simulink model "AGTF30SysDyn_PExPIn"  (R2021b)
settings: Solver=ode4  StartTime=0.0  StopTime=MWS.In.tend  FixedStep=MWS.In.Ts  RelTol=1e-3  EnableMultiTasking=on
model workspace: external: MAT-File (data not in the file)
values from neighbouring files (symbols this model uses):
  MWS = setup_initialize(MWS,startPt,SSsolverSP)    [Setup_Simulation.m]    (also in run_AGTF30e_script.m = Setup_Simulation(inputMethod,MWS.In,filename,Mdl,SSsolverSP,)
undefined symbols (not defined in the file or in its folder): DiscIntNeverNeededParam
libraries: Lib_Solve_ModelSource_TMATS x28, Lib_Cntrl_FirstOrderSensor_TMATS x19, simulink x12, Lib_Cntrl_FirstOrderActuator_TMATS x2, Lib_Cntrl_LimitSelect_TMATS x2, Lib_Solve_OuterLoopIntegrator_TMATS x2, Lib_Cntrl_CorrectedSpeed_TMATS x1, Lib_Solve_IterNRSolverJC_TMATS x1
(part 5 of 6)

== system AGTF30SysDyn_PExPIn/Control System/Wf Controller/Controller/Wf Limit Controllers/Accel Controller ==
  Alt : Inport
  MN : Inport  Port=2
  N1cN : Inport  Port=3
  phiEPT : Inport  Port=4
  phiBoost : Inport  Port=5
  Wfmax : Inport  Port=6
  Wfcmd : Inport  Port=7
  ps3 : Inport  Port=8
  Constant : Constant  Value=MWS.In.Options.WfTransientLogic
  Constant1 : Constant  Value=MWS.In.Options.HybridConfig
  Constant2 : Constant
  Constant3 : Constant  Value=-4*MWS.In.Ts
  Constant4 : Constant  Value=MWS.In.Options.TEEM
  Constant5 : Constant
  Constant6 : Constant  Value=1.1/1.03
  Divide1 : Product  Inputs=**
  Divide2 : Product  Inputs=**
  Divide3 : Product  Inputs=*/
  Divide4 : Product  Inputs=**
  Gain2 : Gain  Gain=MWS.Cntrl.WfCntrl.GenAccel.CeilingMultiplier
  Math Function : Math  SaturateOnIntegerOverflow=on
  Memory : Memory  InitialCondition=MWS.Init.IC.Wf
  Multiport Switch : MultiPortSwitch
  RUSched_Boost : Lookup_n-D  NumberOfTableDimensions=5  BreakpointsForDimension1=MWS.Cntrl.WfCntrl.Accel.Boost.RUsch.N1cN_vec  BreakpointsForDimension2=MWS.Cntrl.WfCntrl.Accel.Boost.RUsch.Alt_vec  BreakpointsForDimension3=MWS.Cntrl.WfCntrl.Accel.Boost.RUsch.MN_vec  BreakpointsForDimension4=MWS.Cntrl.WfCntrl.Accel.Boost.RUsch.phiEPT_vec  BreakpointsForDimension5=MWS.Cntrl.WfCntrl.Accel.Boost.RUsch.phiBoost_vec  Table=MWS.Cntrl.WfCntrl.Accel.Boost.RUsch.RU_array  ExtrapMethod=Clip  InternalRulePriority=Speed  RndMeth=Simplest  InputSameDT=on
      settings: InputPortMap=u0,u1,u2,u3,u4
  RUSched_PEx : Lookup_n-D  NumberOfTableDimensions=4  BreakpointsForDimension1=MWS.Cntrl.WfCntrl.Accel.PEx.RUsch.N1cN_vec  BreakpointsForDimension2=MWS.Cntrl.WfCntrl.Accel.PEx.RUsch.Alt_vec  BreakpointsForDimension3=MWS.Cntrl.WfCntrl.Accel.PEx.RUsch.MN_vec  BreakpointsForDimension4=MWS.Cntrl.WfCntrl.Accel.PEx.RUsch.phiEPT_vec  Table=MWS.Cntrl.WfCntrl.Accel.PEx.RUsch.RU_array  ExtrapMethod=Clip  InternalRulePriority=Speed  RndMeth=Simplest  InputSameDT=on
      settings: InputPortMap=u0,u1,u2,u3
  RUSched_STD : Lookup_n-D  NumberOfTableDimensions=4  BreakpointsForDimension1=MWS.Cntrl.WfCntrl.Accel.STD.RUsch.N1cN_vec  BreakpointsForDimension2=MWS.Cntrl.WfCntrl.Accel.STD.RUsch.Alt_vec  BreakpointsForDimension3=MWS.Cntrl.WfCntrl.Accel.STD.RUsch.MN_vec  BreakpointsForDimension4=MWS.Cntrl.WfCntrl.Accel.STD.RUsch.phiEPT_vec  Table=MWS.Cntrl.WfCntrl.Accel.STD.RUsch.RU_array  ExtrapMethod=Clip  InternalRulePriority=Speed  RndMeth=Simplest  InputSameDT=on
      settings: InputPortMap=u0,u1,u2,u3
  Settling Time Lookup : Lookup_n-D  NumberOfTableDimensions=1  BreakpointsForDimension1=MWS.Cntrl.WfCntrl.GenAccel.Alt_vec  BreakpointsForDimension2=MWS.Cntrl.STD.Wf.CntrlLimits.Cntrl.RUmax.Alt_vec  BreakpointsForDimension3=MWS.Cntrl.STD.Wf.CntrlLimits.Cntrl.RUmax.MN_vec  Table=MWS.Cntrl.WfCntrl.GenAccel.ts_vec  ExtrapMethod=Clip  InternalRulePriority=Speed  RndMeth=Simplest  InputSameDT=on
  Sum : Sum  Inputs=|+-
  Sum1 : Sum  Inputs=|+-
  Sum2 : Sum  Inputs=|++
  Switch : Switch  Criteria=u2 > Threshold  Threshold=1.5
  Switch1 : Switch  Criteria=u2 > Threshold  Threshold=0.5
  Wfdmd : Outport  VectorParamsAs1DForOutWhenUnconnected=off
  WfmaxAccel_SP : Outport  Port=2  VectorParamsAs1DForOutWhenUnconnected=off
  wires:
  Gain2/1 -> Sum/1
  Divide2/1 -> Sum2/1
  Switch/1 -> Wfdmd/1, WfmaxAccel_SP/1
  Sum1/1 -> Divide2/1
  Divide3/1 -> Math Function/1
  Settling Time Lookup/1 -> Divide3/2
  Constant3/1 -> Divide3/1
  Alt/1 -> RUSched_Boost/2, RUSched_STD/2, RUSched_PEx/2, Settling Time Lookup/1
  Sum/1 -> Divide2/2
  Math Function/1 -> Sum1/2
  Constant2/1 -> Sum1/1
  Memory/1 -> Sum/2, Sum2/2
  Wfmax/1 -> Gain2/1
  Wfcmd/1 -> Memory/1
  Constant/1 -> Switch/2
  Sum2/1 -> Switch/3
  Constant1/1 -> Multiport Switch/1
  MN/1 -> RUSched_STD/3, RUSched_PEx/3, RUSched_Boost/3
  phiEPT/1 -> RUSched_STD/4, RUSched_PEx/4, RUSched_Boost/4
  phiBoost/1 -> RUSched_Boost/5
  RUSched_STD/1 -> Multiport Switch/2
  RUSched_Boost/1 -> Multiport Switch/3
  RUSched_PEx/1 -> Multiport Switch/4
  ps3/1 -> Divide1/2
  Multiport Switch/1 -> Divide4/2
  Divide1/1 -> Switch/1
  N1cN/1 -> RUSched_PEx/1, RUSched_Boost/1, RUSched_STD/1
  Divide4/1 -> Divide1/1
  Constant4/1 -> Switch1/2
  Constant5/1 -> Switch1/1
  Constant6/1 -> Switch1/3
  Switch1/1 -> Divide4/1

== system AGTF30SysDyn_PExPIn/Control System/Wf Controller/Controller/Wf Limit Controllers/Decel Controller ==
  Alt : Inport
  MN : Inport  Port=2
  N1cN : Inport  Port=3
  phiEPT : Inport  Port=4
  phiBoost : Inport  Port=5
  Wfmin : Inport  Port=6
  Wf : Inport  Port=7
  ps3 : Inport  Port=8
  Compare To Constant : simulink/Logic and Bit Operations/Compare To Constant  relop=>=  const=1.5  OutDataTypeStr=boolean
  Compare To Constant1 : simulink/Logic and Bit Operations/Compare To Constant  relop=<=  const=0.1  OutDataTypeStr=boolean
  Constant : Constant  Value=MWS.In.Options.WfTransientLogic
  Constant1 : Constant  Value=MWS.In.Options.HybridConfig
  Constant2 : Constant
  Constant3 : Constant  Value=-4*MWS.In.Ts
  Constant4 : Constant  Value=MWS.In.Options.EngineEMInt
  Constant5 : Constant  Value=0.95
  Constant6 : Constant
  Constant7 : Constant  Value=0.94
  Divide1 : Product  Inputs=**
  Divide2 : Product  Inputs=**
  Divide3 : Product  Inputs=*/
  Divide4 : Product  Inputs=**
  Gain2 : Gain  Gain=MWS.Cntrl.WfCntrl.GenDecel.FloorMultiplier
  Logical Operator : Logic  AllPortsSameDT=off  OutDataTypeStr=boolean
  Math Function : Math  SaturateOnIntegerOverflow=on
  Memory : Memory  InitialCondition=MWS.Init.IC.Wf
  Multiport Switch : MultiPortSwitch
  RUSched_Boost : Lookup_n-D  NumberOfTableDimensions=5  BreakpointsForDimension1=MWS.Cntrl.WfCntrl.Decel.Boost.RUsch.N1cN_vec  BreakpointsForDimension2=MWS.Cntrl.WfCntrl.Decel.Boost.RUsch.Alt_vec  BreakpointsForDimension3=MWS.Cntrl.WfCntrl.Decel.Boost.RUsch.MN_vec  BreakpointsForDimension4=MWS.Cntrl.WfCntrl.Decel.Boost.RUsch.phiEPT_vec  BreakpointsForDimension5=MWS.Cntrl.WfCntrl.Decel.Boost.RUsch.phiBoost_vec  Table=MWS.Cntrl.WfCntrl.Decel.Boost.RUsch.RU_array  ExtrapMethod=Clip  InternalRulePriority=Speed  RndMeth=Simplest  InputSameDT=on
      settings: InputPortMap=u0,u1,u2,u3,u4
  RUSched_PEx : Lookup_n-D  NumberOfTableDimensions=4  BreakpointsForDimension1=MWS.Cntrl.WfCntrl.Decel.PEx.RUsch.N1cN_vec  BreakpointsForDimension2=MWS.Cntrl.WfCntrl.Decel.PEx.RUsch.Alt_vec  BreakpointsForDimension3=MWS.Cntrl.WfCntrl.Decel.PEx.RUsch.MN_vec  BreakpointsForDimension4=MWS.Cntrl.WfCntrl.Decel.PEx.RUsch.phiEPT_vec  Table=MWS.Cntrl.WfCntrl.Decel.PEx.RUsch.RU_array  ExtrapMethod=Clip  InternalRulePriority=Speed  RndMeth=Simplest  InputSameDT=on
      settings: InputPortMap=u0,u1,u2,u3
  RUSched_STD : Lookup_n-D  NumberOfTableDimensions=4  BreakpointsForDimension1=MWS.Cntrl.WfCntrl.Decel.STD.RUsch.N1cN_vec  BreakpointsForDimension2=MWS.Cntrl.WfCntrl.Decel.STD.RUsch.Alt_vec  BreakpointsForDimension3=MWS.Cntrl.WfCntrl.Decel.STD.RUsch.MN_vec  BreakpointsForDimension4=MWS.Cntrl.WfCntrl.Decel.STD.RUsch.phiEPT_vec  Table=MWS.Cntrl.WfCntrl.Decel.STD.RUsch.RU_array  ExtrapMethod=Clip  InternalRulePriority=Speed  RndMeth=Simplest  InputSameDT=on
      settings: InputPortMap=u0,u1,u2,u3
  Scope : Scope
  Scope1 : Scope
  Settling Time Lookup : Lookup_n-D  NumberOfTableDimensions=1  BreakpointsForDimension1=MWS.Cntrl.WfCntrl.GenDecel.Alt_vec  BreakpointsForDimension2=MWS.Cntrl.STD.Wf.CntrlLimits.Cntrl.RUmax.Alt_vec  BreakpointsForDimension3=MWS.Cntrl.STD.Wf.CntrlLimits.Cntrl.RUmax.MN_vec  Table=MWS.Cntrl.WfCntrl.GenDecel.ts_vec  ExtrapMethod=Clip  InternalRulePriority=Speed  RndMeth=Simplest  InputSameDT=on
  Sum : Sum  Inputs=|+-
  Sum1 : Sum  Inputs=|+-
  Sum2 : Sum  Inputs=|++
  Switch : Switch  Criteria=u2 > Threshold  Threshold=1.5
  Switch1 : Switch  Criteria=u2 > Threshold  Threshold=0.5
  Switch2 : Switch  Criteria=u2 > Threshold  Threshold=1.5
  Wfdmd : Outport  VectorParamsAs1DForOutWhenUnconnected=off
  WfminDecel_SP : Outport  Port=2  VectorParamsAs1DForOutWhenUnconnected=off
  wires:
  Gain2/1 -> Sum/1
  Divide2/1 -> Sum2/1
  Sum/1 -> Divide2/2
  Constant2/1 -> Sum1/1
  Memory/1 -> Sum/2, Sum2/2
  Settling Time Lookup/1 -> Divide3/2
  Math Function/1 -> Sum1/2
  Divide3/1 -> Math Function/1
  Sum1/1 -> Divide2/1
  Constant3/1 -> Divide3/1
  Switch/1 -> WfminDecel_SP/1, Wfdmd/1
  Wf/1 -> Memory/1
  Wfmin/1 -> Gain2/1
  RUSched_PEx/1 -> Multiport Switch/4
  RUSched_STD/1 -> Multiport Switch/2
  Alt/1 -> RUSched_STD/2, RUSched_Boost/2, RUSched_PEx/2, Settling Time Lookup/1
  MN/1 -> RUSched_STD/3, RUSched_Boost/3, RUSched_PEx/3
  phiEPT/1 -> RUSched_Boost/4, RUSched_PEx/4, RUSched_STD/4
  phiBoost/1 -> RUSched_Boost/5
  Constant1/1 -> Switch2/2, Multiport Switch/1
  Constant/1 -> Switch/2
  RUSched_Boost/1 -> Multiport Switch/3
  Sum2/1 -> Switch/3
  ps3/1 -> Divide1/2
  Multiport Switch/1 -> Divide4/2
  Divide1/1 -> Switch/1
  N1cN/1 -> Compare To Constant1/1, RUSched_Boost/1, RUSched_PEx/1, RUSched_STD/1
  Constant6/1 -> Switch1/3
  Divide4/1 -> Divide1/1
  Switch1/1 -> Scope1/1, Divide4/1
  Constant4/1 -> Compare To Constant/1
  Compare To Constant/1 -> Logical Operator/2
  Logical Operator/1 -> Scope/1, Switch1/2
  Compare To Constant1/1 -> Logical Operator/1
  Constant5/1 -> Switch2/3
  Constant7/1 -> Switch2/1
  Switch2/1 -> Switch1/1

== system AGTF30SysDyn_PExPIn/Control System/Electric Machine Controllers/VEATE EM Controllers/Base Power/Base Power - Boost and PEx/Boost PEx - HC LR CS ==
  note: HP EM
  note: LP EM
  note: HP - CARRIER, LP - RING, COUPLING - SUN
  note: COUPLING EM
  PwrL_Base : Inport
  PwrH_Base : Inport  Port=2
  NS : Inport  Port=3
  NR : Inport  Port=4
  NC : Inport  Port=5
  Abs : Abs
  Abs1 : Abs
  Abs2 : Abs
  CTrqCS : Constant  Value=MWS.Shaft.PGB.TrqCoeff.CTrqCS
  CTrqRS : Constant  Value=MWS.Shaft.PGB.TrqCoeff.CTrqRS
  CTrqRS1 : Constant  Value=MWS.Shaft.PGB.TrqCoeff.CTrqRS
  Divide : Product  Inputs=**/
  Divide1 : Product  Inputs=*/
  Divide{2..3,6..7,10..11} (6 alike) : Product  Inputs=**
  Divide4 : Product  Inputs=*/
  Divide5 : Product  Inputs=***
  Divide8 : Product  Inputs=*/
  Divide9 : Product  Inputs=***
  Gain1 : Gain  Gain=1/5252.113
  Gain15 : Gain  Gain=1/MWS.Shaft.PGB.Sun.GR_gb %GR_gb = Ngb/Nem
  Gain2 : Gain  Gain=1/5252.113
  Gain3 : Gain  Gain=1/MWS.Shaft.PGB.Ring.GR_gb %GR_gb = Ngb/Nem
  Gain4 : Gain  Gain=1/5252.113
  Gain5 : Gain  Gain=1/MWS.Shaft.PGB.Sun.GR_gb %GR_gb = Ngb/Nem
  MinMax : MinMax
  MinMax1 : MinMax
  MinMax2 : MinMax
  Mux1 : Mux  Inputs=3
  Mux2 : Mux  Inputs=3
  Mux3 : Mux  Inputs=3
  PwrMax_Base : Constant  Value=MWS.Cntrl.EMS.PwrMax_Base
  PwrMax_Base1 : Constant  Value=MWS.Cntrl.EMR.PwrMax_Base
  PwrMax_Base2 : Constant  Value=MWS.Cntrl.EMC.PwrMax_Base
  Sign : Signum
  Sign1 : Signum
  Sign2 : Signum
  Sum : Sum  Inputs=|+-
  Sum1 : Sum  Inputs=|-+
  TrqMax_Base : Constant  Value=MWS.Cntrl.EMS.TrqMax_Base
  TrqMax_Base1 : Constant  Value=MWS.Cntrl.EMR.TrqMax_Base
  TrqMax_Base2 : Constant  Value=MWS.Cntrl.EMC.TrqMax_Base
  Zero : Constant  Value=0
  PemS_Base : Outport
  PemR_Base : Outport  Port=2
  PemC_Base : Outport  Port=3
  PemP_Base : Outport  Port=4
  wires:
  Zero/1 -> PemP_Base/1
  PwrH_Base/1 -> Sum1/2
  Divide9/1 -> Sum1/1
  CTrqRS/1 -> Divide/3
  CTrqRS1/1 -> Divide5/3
  Sign2/1 -> Divide11/1
  CTrqCS/1 -> Divide9/3
  Sign/1 -> Divide2/1
  Abs1/1 -> MinMax1/1
  MinMax2/1 -> Divide11/2
  NS/1 -> [NS], Divide1/1
  TrqMax_Base1/1 -> Divide6/1
  Divide6/1 -> Gain2/1
  Divide11/1 -> PemC_Base/1
  Gain2/1 -> Mux2/3
  Mux1/1 -> Abs/1
  PwrMax_Base/1 -> Mux1/2
  [NR] -> Divide4/1
  NR/1 -> [NR], Divide1/2
  Abs2/1 -> MinMax2/1
  [NS] -> Divide4/2
  [NR] -> Gain3/1
  Gain15/1 -> Divide3/2
  [NS] -> Divide8/2
  Divide5/1 -> Sum/2
  Sum1/1 -> Sign2/1, Mux3/1
  Gain1/1 -> Mux1/3
  PwrL_Base/1 -> Divide/1, [PwrL_Base]
  Divide8/1 -> Divide9/2
  Gain3/1 -> Divide6/2
  Gain4/1 -> Mux3/3
  [PemS_Base] -> Divide9/1
  Divide4/1 -> Divide5/2
  [NS] -> Gain15/1
  Divide2/1 -> [PemS_Base], PemS_Base/1
  [PwrL_Base] -> Sum/1
  Divide10/1 -> Gain4/1
  TrqMax_Base2/1 -> Divide10/1
  MinMax/1 -> Divide2/2
  Divide/1 -> Sign/1, Mux1/1  "Power to LP from Coupling"
  Mux3/1 -> Abs2/1
  NC/1 -> Divide8/1, Gain5/1
  Divide7/1 -> PemR_Base/1
  PwrMax_Base2/1 -> Mux3/2
  Gain5/1 -> Divide10/2
  PwrMax_Base1/1 -> Mux2/2
  Abs/1 -> MinMax/1
  MinMax1/1 -> Divide7/2
  Sum/1 -> Sign1/1, Mux2/1  "Power to LP from LP EM"
  [PemS_Base] -> Divide5/1
  Divide1/1 -> Divide/2
  Sign1/1 -> Divide7/1
  Divide3/1 -> Gain1/1
  TrqMax_Base/1 -> Divide3/1
  Mux2/1 -> Abs1/1

== system AGTF30SysDyn_PExPIn/Control System/Electric Machine Controllers/VEATE EM Controllers/Base Power/Base Power - Boost and PEx/Boost PEx - HC LS CR ==
  note: HP EM
  note: LP EM
  note: HP - CARRIER, LP - SUN, COUPLING - RING
  note: COUPLING EM
  PwrL_Base : Inport
  PwrH_Base : Inport  Port=2
  NS : Inport  Port=3
  NR : Inport  Port=4
  NC : Inport  Port=5
  Abs : Abs
  Abs1 : Abs
  Abs2 : Abs
  CTrqCR : Constant  Value=MWS.Shaft.PGB.TrqCoeff.CTrqCR
  CTrqSR : Constant  Value=MWS.Shaft.PGB.TrqCoeff.CTrqSR
  CTrqSR1 : Constant  Value=MWS.Shaft.PGB.TrqCoeff.CTrqSR
  Divide : Product  Inputs=**/
  Divide1 : Product  Inputs=*/
  Divide{2..3,6..7,10..11} (6 alike) : Product  Inputs=**
  Divide4 : Product  Inputs=*/
  Divide5 : Product  Inputs=***
  Divide8 : Product  Inputs=*/
  Divide9 : Product  Inputs=***
  Gain1 : Gain  Gain=1/5252.113
  Gain15 : Gain  Gain=1/MWS.Shaft.PGB.Ring.GR_gb %GR_gb = Ngb/Nem
  Gain2 : Gain  Gain=1/5252.113
  Gain3 : Gain  Gain=1/MWS.Shaft.PGB.Sun.GR_gb %GR_gb = Ngb/Nem
  Gain4 : Gain  Gain=1/5252.113
  Gain5 : Gain  Gain=1/MWS.Shaft.PGB.Carrier.GR_gb %GR_gb = Ngb/Nem
  MinMax : MinMax
  MinMax1 : MinMax
  MinMax2 : MinMax
  Mux1 : Mux  Inputs=3
  Mux2 : Mux  Inputs=3
  Mux3 : Mux  Inputs=3
  PwrMax_Base : Constant  Value=MWS.Cntrl.EMR.PwrMax_Base
  PwrMax_Base1 : Constant  Value=MWS.Cntrl.EMS.PwrMax_Base
  PwrMax_Base2 : Constant  Value=MWS.Cntrl.EMC.PwrMax_Base
  Sign : Signum
  Sign1 : Signum
  Sign2 : Signum
  Sum : Sum  Inputs=|+-
  Sum1 : Sum  Inputs=|-+
  TrqMax_Base : Constant  Value=MWS.Cntrl.EMR.TrqMax_Base
  TrqMax_Base1 : Constant  Value=MWS.Cntrl.EMS.TrqMax_Base
  TrqMax_Base2 : Constant  Value=MWS.Cntrl.EMC.TrqMax_Base
  Zero : Constant  Value=0
  PemS_Base : Outport
  PemR_Base : Outport  Port=2
  PemC_Base : Outport  Port=3
  PemP_Base : Outport  Port=4
  wires:
  [NR] -> Divide4/2
  [NS] -> Divide4/1
  Zero/1 -> PemP_Base/1
  PwrH_Base/1 -> Sum1/2
  Divide9/1 -> Sum1/1
  CTrqSR/1 -> Divide/3
  CTrqSR1/1 -> Divide5/3
  Sign2/1 -> Divide11/1
  CTrqCR/1 -> Divide9/3
  Sign/1 -> Divide2/1
  Abs1/1 -> MinMax1/1
  MinMax2/1 -> Divide11/2
  NR/1 -> [NR], Divide1/1
  TrqMax_Base1/1 -> Divide6/1
  Divide6/1 -> Gain2/1
  Divide11/1 -> PemC_Base/1
  Gain2/1 -> Mux2/3
  Mux1/1 -> Abs/1
  PwrMax_Base/1 -> Mux1/2
  NS/1 -> Divide1/2, [NS]
  Abs2/1 -> MinMax2/1
  [NS] -> Gain3/1
  Gain15/1 -> Divide3/2
  [NR] -> Divide8/2
  Divide5/1 -> Sum/2
  Sum1/1 -> Sign2/1, Mux3/1
  Gain1/1 -> Mux1/3
  PwrL_Base/1 -> Divide/1, [PwrL_Base]
  Divide8/1 -> Divide9/2
  Gain3/1 -> Divide6/2
  Gain4/1 -> Mux3/3
  [PemR_Base] -> Divide9/1
  Divide4/1 -> Divide5/2
  [NR] -> Gain15/1
  Divide2/1 -> PemR_Base/1, [PemR_Base]
  [PwrL_Base] -> Sum/1
  Divide10/1 -> Gain4/1
  TrqMax_Base2/1 -> Divide10/1
  MinMax/1 -> Divide2/2
  Divide/1 -> Sign/1, Mux1/1  "Power to LP from Coupling"
  Mux3/1 -> Abs2/1
  NC/1 -> Divide8/1, Gain5/1
  Divide7/1 -> PemS_Base/1
  PwrMax_Base2/1 -> Mux3/2
  Gain5/1 -> Divide10/2
  PwrMax_Base1/1 -> Mux2/2
  Abs/1 -> MinMax/1
  MinMax1/1 -> Divide7/2
  Sum/1 -> Sign1/1, Mux2/1  "Power to LP from LP EM"
  [PemR_Base] -> Divide5/1
  Divide1/1 -> Divide/2
  Sign1/1 -> Divide7/1
  Divide3/1 -> Gain1/1
  TrqMax_Base/1 -> Divide3/1
  Mux2/1 -> Abs1/1

== system AGTF30SysDyn_PExPIn/Control System/Electric Machine Controllers/VEATE EM Controllers/Base Power/Base Power - Boost and PEx/Boost PEx - HR LC CS  ==
  note: COUPLING EM
  note: HP - RING, LP - CARRIER, COUPLING - SUN
  note: LP EM
  note: HP EM
  PwrL_Base : Inport
  PwrH_Base : Inport  Port=2
  NS : Inport  Port=3
  NR : Inport  Port=4
  NC : Inport  Port=5
  Abs : Abs
  Abs1 : Abs
  Abs2 : Abs
  CTrqCS : Constant  Value=MWS.Shaft.PGB.TrqCoeff.CTrqCS
  CTrqCS1 : Constant  Value=MWS.Shaft.PGB.TrqCoeff.CTrqCS
  CTrqRS : Constant  Value=MWS.Shaft.PGB.TrqCoeff.CTrqRS
  Divide : Product  Inputs=**/
  Divide1 : Product  Inputs=*/
  Divide{2..3,6..7,10..11} (6 alike) : Product  Inputs=**
  Divide4 : Product  Inputs=*/
  Divide5 : Product  Inputs=***
  Divide8 : Product  Inputs=*/
  Divide9 : Product  Inputs=***
  Gain1 : Gain  Gain=1/5252.113
  Gain15 : Gain  Gain=1/MWS.Shaft.PGB.Sun.GR_gb %GR_gb = Ngb/Nem
  Gain2 : Gain  Gain=1/5252.113
  Gain3 : Gain  Gain=1/MWS.Shaft.PGB.Carrier.GR_gb %GR_gb = Ngb/Nem
  Gain4 : Gain  Gain=1/5252.113
  Gain5 : Gain  Gain=1/MWS.Shaft.PGB.Ring.GR_gb %GR_gb = Ngb/Nem
  MinMax : MinMax
  MinMax1 : MinMax
  MinMax2 : MinMax
  Mux1 : Mux  Inputs=3
  Mux2 : Mux  Inputs=3
  Mux3 : Mux  Inputs=3
  PwrMax_Base : Constant  Value=MWS.Cntrl.EMS.PwrMax_Base
  PwrMax_Base1 : Constant  Value=MWS.Cntrl.EMC.PwrMax_Base
  PwrMax_Base2 : Constant  Value=MWS.Cntrl.EMR.PwrMax_Base
  Sign : Signum
  Sign1 : Signum
  Sign2 : Signum
  Sum : Sum  Inputs=|+-
  Sum1 : Sum  Inputs=|-+
  TrqMax_Base : Constant  Value=MWS.Cntrl.EMS.TrqMax_Base
  TrqMax_Base1 : Constant  Value=MWS.Cntrl.EMC.TrqMax_Base
  TrqMax_Base2 : Constant  Value=MWS.Cntrl.EMR.TrqMax_Base
  Zero : Constant  Value=0
  PemS_Base : Outport
  PemR_Base : Outport  Port=2
  PemC_Base : Outport  Port=3
  PemP_Base : Outport  Port=4
  wires:
  Mux2/1 -> Abs1/1
  TrqMax_Base/1 -> Divide3/1
  Divide3/1 -> Gain1/1
  Sign1/1 -> Divide7/1
  Divide1/1 -> Divide/2
  [PemS_Base] -> Divide5/1
  Sum/1 -> Mux2/1, Sign1/1  "Power to LP from LP EM"
  MinMax1/1 -> Divide7/2
  Abs/1 -> MinMax/1
  PwrMax_Base1/1 -> Mux2/2
  Gain5/1 -> Divide10/2
  PwrMax_Base2/1 -> Mux3/2
  Divide7/1 -> PemC_Base/1
  NR/1 -> Gain5/1, Divide8/1
  Mux3/1 -> Abs2/1
  Divide/1 -> Mux1/1, Sign/1  "Power to LP from Coupling"
  MinMax/1 -> Divide2/2
  TrqMax_Base2/1 -> Divide10/1
  Divide10/1 -> Gain4/1
  [PwrL_Base] -> Sum/1
  Divide2/1 -> PemS_Base/1, [PemS_Base]
  [NS] -> Gain15/1
  Divide4/1 -> Divide5/2
  [PemS_Base] -> Divide9/1
  Gain4/1 -> Mux3/3
  Gain3/1 -> Divide6/2
  Divide8/1 -> Divide9/2
  PwrL_Base/1 -> [PwrL_Base], Divide/1
  Gain1/1 -> Mux1/3
  Sum1/1 -> Mux3/1, Sign2/1
  Divide5/1 -> Sum/2
  [NS] -> Divide8/2
  Gain15/1 -> Divide3/2
  [NC] -> Gain3/1
  [NS] -> Divide4/2
  Abs2/1 -> MinMax2/1
  NC/1 -> Divide1/2, [NC]
  [NC] -> Divide4/1
  PwrMax_Base/1 -> Mux1/2
  Mux1/1 -> Abs/1
  Gain2/1 -> Mux2/3
  Divide11/1 -> PemR_Base/1
  Divide6/1 -> Gain2/1
  TrqMax_Base1/1 -> Divide6/1
  NS/1 -> Divide1/1, [NS]
  MinMax2/1 -> Divide11/2
  Abs1/1 -> MinMax1/1
  Sign/1 -> Divide2/1
  CTrqRS/1 -> Divide9/3
  Sign2/1 -> Divide11/1
  CTrqCS1/1 -> Divide5/3
  CTrqCS/1 -> Divide/3
  Divide9/1 -> Sum1/1
  PwrH_Base/1 -> Sum1/2
  Zero/1 -> PemP_Base/1

== system AGTF30SysDyn_PExPIn/Control System/Electric Machine Controllers/VEATE EM Controllers/Base Power/Base Power - Boost and PEx/Boost PEx - HR LS CC ==
  note: COUPLING EM
  note: HP - RING, LP - SUN, COUPLING - CARRIER
  note: LP EM
  note: HP EM
  PwrL_Base : Inport
  PwrH_Base : Inport  Port=2
  NS : Inport  Port=3
  NR : Inport  Port=4
  NC : Inport  Port=5
  Abs : Abs
  Abs1 : Abs
  Abs2 : Abs
  CTrqRC : Constant  Value=MWS.Shaft.PGB.TrqCoeff.CTrqRC
  CTrqSC : Constant  Value=MWS.Shaft.PGB.TrqCoeff.CTrqSC
  CTrqSC1 : Constant  Value=MWS.Shaft.PGB.TrqCoeff.CTrqSC
  Divide : Product  Inputs=**/
  Divide1 : Product  Inputs=*/
  Divide{2..3,6..7,10..11} (6 alike) : Product  Inputs=**
  Divide4 : Product  Inputs=*/
  Divide5 : Product  Inputs=***
  Divide8 : Product  Inputs=*/
  Divide9 : Product  Inputs=***
  Gain1 : Gain  Gain=1/5252.113
  Gain15 : Gain  Gain=1/MWS.Shaft.PGB.Carrier.GR_gb %GR_gb = Ngb/Nem
  Gain2 : Gain  Gain=1/5252.113
  Gain3 : Gain  Gain=1/MWS.Shaft.PGB.Sun.GR_gb %GR_gb = Ngb/Nem
  Gain4 : Gain  Gain=1/5252.113
  Gain5 : Gain  Gain=1/MWS.Shaft.PGB.Ring.GR_gb %GR_gb = Ngb/Nem
  MinMax : MinMax
  MinMax1 : MinMax
  MinMax2 : MinMax
  Mux1 : Mux  Inputs=3
  Mux2 : Mux  Inputs=3
  Mux3 : Mux  Inputs=3
  PwrMax_Base : Constant  Value=MWS.Cntrl.EMC.PwrMax_Base
  PwrMax_Base1 : Constant  Value=MWS.Cntrl.EMS.PwrMax_Base
  PwrMax_Base2 : Constant  Value=MWS.Cntrl.EMR.PwrMax_Base
  Sign : Signum
  Sign1 : Signum
  Sign2 : Signum
  Sum : Sum  Inputs=|+-
  Sum1 : Sum  Inputs=|-+
  TrqMax_Base : Constant  Value=MWS.Cntrl.EMC.TrqMax_Base
  TrqMax_Base1 : Constant  Value=MWS.Cntrl.EMS.TrqMax_Base
  TrqMax_Base2 : Constant  Value=MWS.Cntrl.EMR.TrqMax_Base
  Zero : Constant  Value=0
  PemS_Base : Outport
  PemR_Base : Outport  Port=2
  PemC_Base : Outport  Port=3
  PemP_Base : Outport  Port=4
  wires:
  Mux2/1 -> Abs1/1
  TrqMax_Base/1 -> Divide3/1
  Divide3/1 -> Gain1/1
  Sign1/1 -> Divide7/1
  Divide1/1 -> Divide/2
  [PemC_Base] -> Divide5/1
  Sum/1 -> Mux2/1, Sign1/1  "Power to LP from LP EM"
  MinMax1/1 -> Divide7/2
  Abs/1 -> MinMax/1
  PwrMax_Base1/1 -> Mux2/2
  Gain5/1 -> Divide10/2
  PwrMax_Base2/1 -> Mux3/2
  Divide7/1 -> PemS_Base/1
  NR/1 -> Gain5/1, Divide8/1
  Mux3/1 -> Abs2/1
  Divide/1 -> Mux1/1, Sign/1  "Power to LP from Coupling"
  MinMax/1 -> Divide2/2
  TrqMax_Base2/1 -> Divide10/1
  Divide10/1 -> Gain4/1
  [PwrL_Base] -> Sum/1
  Divide2/1 -> PemC_Base/1, [PemC_Base]
  [NC] -> Gain15/1
  Divide4/1 -> Divide5/2
  [PemC_Base] -> Divide9/1
  Gain4/1 -> Mux3/3
  Gain3/1 -> Divide6/2
  Divide8/1 -> Divide9/2
  PwrL_Base/1 -> [PwrL_Base], Divide/1
  Gain1/1 -> Mux1/3
  Sum1/1 -> Mux3/1, Sign2/1
  Divide5/1 -> Sum/2
  [NC] -> Divide8/2
  Gain15/1 -> Divide3/2
  [NS] -> Gain3/1
  Abs2/1 -> MinMax2/1
  NS/1 -> [NS], Divide1/2
  PwrMax_Base/1 -> Mux1/2
  Mux1/1 -> Abs/1
  Gain2/1 -> Mux2/3
  Divide11/1 -> PemR_Base/1
  Divide6/1 -> Gain2/1
  TrqMax_Base1/1 -> Divide6/1
  NC/1 -> Divide1/1, [NC]
  MinMax2/1 -> Divide11/2
  Abs1/1 -> MinMax1/1
  Sign/1 -> Divide2/1
  CTrqRC/1 -> Divide9/3
  Sign2/1 -> Divide11/1
  CTrqSC1/1 -> Divide5/3
  CTrqSC/1 -> Divide/3
  Divide9/1 -> Sum1/1
  PwrH_Base/1 -> Sum1/2
  Zero/1 -> PemP_Base/1
  [NS] -> Divide4/1
  [NC] -> Divide4/2

== system AGTF30SysDyn_PExPIn/Control System/Electric Machine Controllers/VEATE EM Controllers/Base Power/Base Power - Boost and PEx/Boost PEx - HS LC CR ==
  note: HP EM
  note: LP EM
  note: HP - SUN, LP - CARRIER, COUPLING - RING
  note: COUPLING EM
  PwrL_Base : Inport
  PwrH_Base : Inport  Port=2
  NS : Inport  Port=3
  NR : Inport  Port=4
  NC : Inport  Port=5
  Abs : Abs
  Abs1 : Abs
  Abs2 : Abs
  CTrqCR : Constant  Value=MWS.Shaft.PGB.TrqCoeff.CTrqCR
  CTrqCR1 : Constant  Value=MWS.Shaft.PGB.TrqCoeff.CTrqCR
  CTrqSR : Constant  Value=MWS.Shaft.PGB.TrqCoeff.CTrqSR
  Divide : Product  Inputs=**/
  Divide1 : Product  Inputs=*/
  Divide{2..3,6..7,10..11} (6 alike) : Product  Inputs=**
  Divide4 : Product  Inputs=*/
  Divide5 : Product  Inputs=***
  Divide8 : Product  Inputs=*/
  Divide9 : Product  Inputs=***
  Gain1 : Gain  Gain=1/5252.113
  Gain15 : Gain  Gain=1/MWS.Shaft.PGB.Ring.GR_gb %GR_gb = Ngb/Nem
  Gain2 : Gain  Gain=1/5252.113
  Gain3 : Gain  Gain=1/MWS.Shaft.PGB.Carrier.GR_gb %GR_gb = Ngb/Nem
  Gain4 : Gain  Gain=1/5252.113
  Gain5 : Gain  Gain=1/MWS.Shaft.PGB.Sun.GR_gb %GR_gb = Ngb/Nem
  MinMax : MinMax
  MinMax1 : MinMax
  MinMax2 : MinMax
  Mux1 : Mux  Inputs=3
  Mux2 : Mux  Inputs=3
  Mux3 : Mux  Inputs=3
  PwrMax_Base : Constant  Value=MWS.Cntrl.EMR.PwrMax_Base
  PwrMax_Base1 : Constant  Value=MWS.Cntrl.EMC.PwrMax_Base
  PwrMax_Base2 : Constant  Value=MWS.Cntrl.EMS.PwrMax_Base
  Sign : Signum
  Sign1 : Signum
  Sign2 : Signum
  Sum : Sum  Inputs=|+-
  Sum1 : Sum  Inputs=|-+
  TrqMax_Base : Constant  Value=MWS.Cntrl.EMR.TrqMax_Base
  TrqMax_Base1 : Constant  Value=MWS.Cntrl.EMC.TrqMax_Base
  TrqMax_Base2 : Constant  Value=MWS.Cntrl.EMS.TrqMax_Base
  Zero : Constant  Value=0
  PemS_Base : Outport
  PemR_Base : Outport  Port=2
  PemC_Base : Outport  Port=3
  PemP_Base : Outport  Port=4
  wires:
  Zero/1 -> PemP_Base/1
  PwrH_Base/1 -> Sum1/2
  Divide9/1 -> Sum1/1
  CTrqCR/1 -> Divide/3
  CTrqCR1/1 -> Divide5/3
  Sign2/1 -> Divide11/1
  CTrqSR/1 -> Divide9/3
  Sign/1 -> Divide2/1
  Abs1/1 -> MinMax1/1
  MinMax2/1 -> Divide11/2
  NR/1 -> [NR], Divide1/1
  TrqMax_Base1/1 -> Divide6/1
  Divide6/1 -> Gain2/1
  Divide11/1 -> PemS_Base/1
  Gain2/1 -> Mux2/3
  Mux1/1 -> Abs/1
  PwrMax_Base/1 -> Mux1/2
  [NC] -> Divide4/1
  NC/1 -> [NC], Divide1/2
  Abs2/1 -> MinMax2/1
  [NR] -> Divide4/2
  [NC] -> Gain3/1
  Gain15/1 -> Divide3/2
  [NR] -> Divide8/2
  Divide5/1 -> Sum/2
  Sum1/1 -> Sign2/1, Mux3/1
  Gain1/1 -> Mux1/3
  PwrL_Base/1 -> Divide/1, [PwrL_Base]
  Divide8/1 -> Divide9/2
  Gain3/1 -> Divide6/2
  Gain4/1 -> Mux3/3
  [PemR_Base] -> Divide9/1
  Divide4/1 -> Divide5/2
  [NR] -> Gain15/1
  Divide2/1 -> [PemR_Base], PemR_Base/1
  [PwrL_Base] -> Sum/1
  Divide10/1 -> Gain4/1
  TrqMax_Base2/1 -> Divide10/1
  MinMax/1 -> Divide2/2
  Divide/1 -> Sign/1, Mux1/1  "Power to LP from Coupling"
  Mux3/1 -> Abs2/1
  NS/1 -> Divide8/1, Gain5/1
  Divide7/1 -> PemC_Base/1
  PwrMax_Base2/1 -> Mux3/2
  Gain5/1 -> Divide10/2
  PwrMax_Base1/1 -> Mux2/2
  Abs/1 -> MinMax/1
  MinMax1/1 -> Divide7/2
  Sum/1 -> Sign1/1, Mux2/1  "Power to LP from LP EM"
  [PemR_Base] -> Divide5/1
  Divide1/1 -> Divide/2
  Sign1/1 -> Divide7/1
  Divide3/1 -> Gain1/1
  TrqMax_Base/1 -> Divide3/1
  Mux2/1 -> Abs1/1

== system AGTF30SysDyn_PExPIn/Control System/Electric Machine Controllers/VEATE EM Controllers/Base Power/Base Power - Boost and PEx/Boost PEx - HS LR CC ==
  note: COUPLING EM
  note: HP - SUN, LP - RING, COUPLING - CARRIER
  note: LP EM
  note: HP EM
  PwrL_Base : Inport
  PwrH_Base : Inport  Port=2
  NS : Inport  Port=3
  NR : Inport  Port=4
  NC : Inport  Port=5
  Abs : Abs
  Abs1 : Abs
  Abs2 : Abs
  CTrqRC : Constant  Value=MWS.Shaft.PGB.TrqCoeff.CTrqRC
  CTrqRC1 : Constant  Value=MWS.Shaft.PGB.TrqCoeff.CTrqRC
  CTrqSC1 : Constant  Value=MWS.Shaft.PGB.TrqCoeff.CTrqSC
  Divide : Product  Inputs=**/
  Divide1 : Product  Inputs=*/
  Divide{2..3,6..7,10..11} (6 alike) : Product  Inputs=**
  Divide4 : Product  Inputs=*/
  Divide5 : Product  Inputs=***
  Divide8 : Product  Inputs=*/
  Divide9 : Product  Inputs=***
  Gain1 : Gain  Gain=1/5252.113
  Gain15 : Gain  Gain=1/MWS.Shaft.PGB.Carrier.GR_gb %GR_gb = Ngb/Nem
  Gain2 : Gain  Gain=1/5252.113
  Gain3 : Gain  Gain=1/MWS.Shaft.PGB.Ring.GR_gb %GR_gb = Ngb/Nem
  Gain4 : Gain  Gain=1/5252.113
  Gain5 : Gain  Gain=1/MWS.Shaft.PGB.Sun.GR_gb %GR_gb = Ngb/Nem
  MinMax : MinMax
  MinMax1 : MinMax
  MinMax2 : MinMax
  Mux1 : Mux  Inputs=3
  Mux2 : Mux  Inputs=3
  Mux3 : Mux  Inputs=3
  PwrMax_Base : Constant  Value=MWS.Cntrl.EMC.PwrMax_Base
  PwrMax_Base1 : Constant  Value=MWS.Cntrl.EMR.PwrMax_Base
  PwrMax_Base2 : Constant  Value=MWS.Cntrl.EMS.PwrMax_Base
  Sign : Signum
  Sign1 : Signum
  Sign2 : Signum
  Sum : Sum  Inputs=|+-
  Sum1 : Sum  Inputs=|-+
  TrqMax_Base : Constant  Value=MWS.Cntrl.EMC.TrqMax_Base
  TrqMax_Base1 : Constant  Value=MWS.Cntrl.EMR.TrqMax_Base
  TrqMax_Base2 : Constant  Value=MWS.Cntrl.EMS.TrqMax_Base
  Zero : Constant  Value=0
  PemS_Base : Outport
  PemR_Base : Outport  Port=2
  PemC_Base : Outport  Port=3
  PemP_Base : Outport  Port=4
  wires:
  Mux2/1 -> Abs1/1
  TrqMax_Base/1 -> Divide3/1
  Divide3/1 -> Gain1/1
  Sign1/1 -> Divide7/1
  Divide1/1 -> Divide/2
  [PemC_Base] -> Divide5/1
  Sum/1 -> Mux2/1, Sign1/1  "Power to LP from LP EM"
  MinMax1/1 -> Divide7/2
  Abs/1 -> MinMax/1
  PwrMax_Base1/1 -> Mux2/2
  Gain5/1 -> Divide10/2
  PwrMax_Base2/1 -> Mux3/2
  Divide7/1 -> PemR_Base/1
  NS/1 -> Gain5/1, Divide8/1
  Mux3/1 -> Abs2/1
  Divide/1 -> Mux1/1, Sign/1  "Power to LP from Coupling"
  MinMax/1 -> Divide2/2
  TrqMax_Base2/1 -> Divide10/1
  Divide10/1 -> Gain4/1
  [PwrL_Base] -> Sum/1
  Divide2/1 -> PemC_Base/1, [PemC_Base]
  [NC] -> Gain15/1
  Divide4/1 -> Divide5/2
  [PemC_Base] -> Divide9/1
  Gain4/1 -> Mux3/3
  Gain3/1 -> Divide6/2
  Divide8/1 -> Divide9/2
  PwrL_Base/1 -> [PwrL_Base], Divide/1
  Gain1/1 -> Mux1/3
  Sum1/1 -> Mux3/1, Sign2/1
  Divide5/1 -> Sum/2
  [NC] -> Divide8/2
  Gain15/1 -> Divide3/2
  [NR] -> Gain3/1
  [NR] -> Divide4/1
  Abs2/1 -> MinMax2/1
  NR/1 -> [NR], Divide1/2
  [NC] -> Divide4/2
  PwrMax_Base/1 -> Mux1/2
  Mux1/1 -> Abs/1
  Gain2/1 -> Mux2/3
  Divide11/1 -> PemS_Base/1
  Divide6/1 -> Gain2/1
  TrqMax_Base1/1 -> Divide6/1
  NC/1 -> [NC], Divide1/1
  MinMax2/1 -> Divide11/2
  Abs1/1 -> MinMax1/1
  Sign/1 -> Divide2/1
  CTrqSC1/1 -> Divide9/3
  Sign2/1 -> Divide11/1
  CTrqRC1/1 -> Divide5/3
  CTrqRC/1 -> Divide/3
  Divide9/1 -> Sum1/1
  PwrH_Base/1 -> Sum1/2
  Zero/1 -> PemP_Base/1

== system AGTF30SysDyn_PExPIn/Control System/Electric Machine Controllers/VEATE EM Controllers/Base Power/Base Power - Standard/Standard - HC ==
  note: HP EM
  note: LP EM / COUPLING EM
  note: HP - CARRIER
  note: COUPLING EM / LP EM
  PwrH_Base : Inport
  NS : Inport  Port=2
  Abs2 : Abs
  Divide10 : Product  Inputs=**
  Divide11 : Product  Inputs=**
  Gain4 : Gain  Gain=1/5252.113
  Gain5 : Gain  Gain=1/MWS.Shaft.PGB.Carrier.GR_gb %GR_gb = Ngb/Nem
  MinMax2 : MinMax
  Mux3 : Mux  Inputs=3
  PwrMax_Base2 : Constant  Value=MWS.Cntrl.EMC.PwrMax_Base
  Sign2 : Signum
  TrqMax_Base2 : Constant  Value=MWS.Cntrl.EMC.TrqMax_Base
  Zero : Constant  Value=0
  Zero1 : Constant  Value=0
  Zero2 : Constant  Value=0
  PemS_Base : Outport
  PemR_Base : Outport  Port=2
  PemC_Base : Outport  Port=3
  PemP_Base : Outport  Port=4
  wires:
  Zero/1 -> PemP_Base/1
  Sign2/1 -> Divide11/1
  MinMax2/1 -> Divide11/2
  Divide11/1 -> PemC_Base/1
  Abs2/1 -> MinMax2/1
  PwrH_Base/1 -> Mux3/1, Sign2/1
  Gain4/1 -> Mux3/3
  Zero1/1 -> PemR_Base/1
  Divide10/1 -> Gain4/1
  TrqMax_Base2/1 -> Divide10/1
  Mux3/1 -> Abs2/1
  NS/1 -> Gain5/1
  Zero2/1 -> PemS_Base/1
  PwrMax_Base2/1 -> Mux3/2
  Gain5/1 -> Divide10/2

== system AGTF30SysDyn_PExPIn/Control System/Electric Machine Controllers/VEATE EM Controllers/Base Power/Base Power - Standard/Standard - HR ==
  note: COUPLING EM / LP EM
  note: HP - RING
  note: LP EM / COUPLING EM
  note: HP EM
  PwrH_Base : Inport
  NR : Inport  Port=2
  Abs2 : Abs
  Divide10 : Product  Inputs=**
  Divide11 : Product  Inputs=**
  Gain4 : Gain  Gain=1/5252.113
  Gain5 : Gain  Gain=1/MWS.Shaft.PGB.Ring.GR_gb %GR_gb = Ngb/Nem
  MinMax2 : MinMax
  Mux3 : Mux  Inputs=3
  PwrMax_Base2 : Constant  Value=MWS.Cntrl.EMR.PwrMax_Base
  Sign2 : Signum
  TrqMax_Base2 : Constant  Value=MWS.Cntrl.EMR.TrqMax_Base
  Zero : Constant  Value=0
  Zero1 : Constant  Value=0
  Zero2 : Constant  Value=0
  PemS_Base : Outport
  PemR_Base : Outport  Port=2
  PemC_Base : Outport  Port=3
  PemP_Base : Outport  Port=4
  wires:
  Gain5/1 -> Divide10/2
  PwrMax_Base2/1 -> Mux3/2
  Zero2/1 -> PemS_Base/1
  NR/1 -> Gain5/1
  Mux3/1 -> Abs2/1
  TrqMax_Base2/1 -> Divide10/1
  Divide10/1 -> Gain4/1
  Zero1/1 -> PemC_Base/1
  Gain4/1 -> Mux3/3
  PwrH_Base/1 -> Sign2/1, Mux3/1
  Abs2/1 -> MinMax2/1
  Divide11/1 -> PemR_Base/1
  MinMax2/1 -> Divide11/2
  Sign2/1 -> Divide11/1
  Zero/1 -> PemP_Base/1

== system AGTF30SysDyn_PExPIn/Control System/Electric Machine Controllers/VEATE EM Controllers/Base Power/Base Power - Standard/Standard - HS ==
  note: HP EM
  note: LP EM / COUPLING EM
  note: HP - SUN
  note: COUPLING EM / LP EM
  PwrH_Base : Inport
  NS : Inport  Port=2
  Abs2 : Abs
  Divide10 : Product  Inputs=**
  Divide11 : Product  Inputs=**
  Gain4 : Gain  Gain=1/5252.113
  Gain5 : Gain  Gain=1/MWS.Shaft.PGB.Sun.GR_gb %GR_gb = Ngb/Nem
  MinMax2 : MinMax
  Mux3 : Mux  Inputs=3
  PwrMax_Base2 : Constant  Value=MWS.Cntrl.EMS.PwrMax_Base
  Sign2 : Signum
  TrqMax_Base2 : Constant  Value=MWS.Cntrl.EMS.TrqMax_Base
  Zero : Constant  Value=0
  Zero1 : Constant  Value=0
  Zero2 : Constant  Value=0
  PemS_Base : Outport
  PemR_Base : Outport  Port=2
  PemC_Base : Outport  Port=3
  PemP_Base : Outport  Port=4
  wires:
  Zero/1 -> PemP_Base/1
  Sign2/1 -> Divide11/1
  MinMax2/1 -> Divide11/2
  Divide11/1 -> PemS_Base/1
  Abs2/1 -> MinMax2/1
  PwrH_Base/1 -> Mux3/1, Sign2/1
  Gain4/1 -> Mux3/3
  Zero1/1 -> PemC_Base/1
  Divide10/1 -> Gain4/1
  TrqMax_Base2/1 -> Divide10/1
  Mux3/1 -> Abs2/1
  NS/1 -> Gain5/1
  Zero2/1 -> PemR_Base/1
  PwrMax_Base2/1 -> Mux3/2
  Gain5/1 -> Divide10/2

== system AGTF30SysDyn_PExPIn/Control System/Electric Machine Controllers/VEATE EM Controllers/TEEM Power/TEEM Power/TEEM - HC LR CS ==
  note: COUPLING EM
  note: HP - CARRIER, LP - RING, COUPLING - SUN
  note: LP EM
  note: HP EM
  Pwr_TEEM : Inport
  NS : Inport  Port=2
  NC : Inport  Port=3
  Abs : Abs
  Abs2 : Abs
  CTrqCS : Constant  Value=MWS.Shaft.PGB.TrqCoeff.CTrqCS
  CTrqCS1 : Constant  Value=MWS.Shaft.PGB.TrqCoeff.CTrqCS
  Divide : Product  Inputs=**/
  Divide1 : Product  Inputs=*/
  Divide{2..3,10..11} (4 alike) : Product  Inputs=**
  Divide8 : Product  Inputs=*/
  Divide9 : Product  Inputs=***
  Gain1 : Gain  Gain=1/5252.113
  Gain15 : Gain  Gain=1/MWS.Shaft.PGB.Sun.GR_gb %GR_gb = Ngb/Nem
  Gain4 : Gain  Gain=1/5252.113
  Gain5 : Gain  Gain=1/MWS.Shaft.PGB.Sun.GR_gb %GR_gb = Ngb/Nem
  MinMax : MinMax
  MinMax2 : MinMax
  Mux1 : Mux  Inputs=3
  Mux3 : Mux  Inputs=3
  PwrMax_Base : Constant  Value=MWS.Cntrl.EMS.PwrMax_TEEM
  PwrMax_Base2 : Constant  Value=MWS.Cntrl.EMC.PwrMax_TEEM
  Sign : Signum
  Sign2 : Signum
  Sum1 : Sum  Inputs=|-+
  TrqMax_Base : Constant  Value=MWS.Cntrl.EMS.TrqMax_TEEM
  TrqMax_Base2 : Constant  Value=MWS.Cntrl.EMC.TrqMax_TEEM
  Zero : Constant  Value=0
  Zero1 : Constant  Value=0
  PemS_TEEM : Outport
  PemR_TEEM : Outport  Port=2
  PemC_TEEM : Outport  Port=3
  PemP_TEEM : Outport  Port=4
  wires:
  TrqMax_Base/1 -> Divide3/1
  Divide3/1 -> Gain1/1
  Divide1/1 -> Divide/2
  Abs/1 -> MinMax/1
  Gain5/1 -> Divide10/2
  PwrMax_Base2/1 -> Mux3/2
  Zero1/1 -> PemR_TEEM/1
  [NC] -> Gain5/1, Divide8/1
  Mux3/1 -> Abs2/1
  Divide/1 -> Mux1/1, Sign/1  "Power to LP from Coupling"
  MinMax/1 -> Divide2/2
  TrqMax_Base2/1 -> Divide10/1
  Divide10/1 -> Gain4/1
  Divide2/1 -> PemS_TEEM/1, [PemS_Base]
  [NS] -> Gain15/1
  [PemS_Base] -> Divide9/1
  Gain4/1 -> Mux3/3
  Divide8/1 -> Divide9/2
  Pwr_TEEM/1 -> [Pwr_TEEM], Divide/1
  Gain1/1 -> Mux1/3
  Sum1/1 -> Mux3/1, Sign2/1
  [NS] -> Divide8/2
  Gain15/1 -> Divide3/2
  Abs2/1 -> MinMax2/1
  NC/1 -> Divide1/2, [NC]
  PwrMax_Base/1 -> Mux1/2
  Mux1/1 -> Abs/1
  Divide11/1 -> PemC_TEEM/1
  NS/1 -> Divide1/1, [NS]
  MinMax2/1 -> Divide11/2
  Sign/1 -> Divide2/1
  CTrqCS/1 -> Divide9/3
  Sign2/1 -> Divide11/1
  CTrqCS1/1 -> Divide/3
  Divide9/1 -> Sum1/1
  [Pwr_TEEM] -> Sum1/2
  Zero/1 -> PemP_TEEM/1

== system AGTF30SysDyn_PExPIn/Control System/Electric Machine Controllers/VEATE EM Controllers/TEEM Power/TEEM Power/TEEM - HC LS CR ==
  note: COUPLING EM
  note: HP - CARRIER, LP - SUN, COUPLING - RING
  note: LP EM
  note: HP EM
  Pwr_TEEM : Inport
  NR : Inport  Port=2
  NC : Inport  Port=3
  Abs : Abs
  Abs2 : Abs
  CTrqCR : Constant  Value=MWS.Shaft.PGB.TrqCoeff.CTrqCR
  CTrqCR1 : Constant  Value=MWS.Shaft.PGB.TrqCoeff.CTrqCR
  Divide : Product  Inputs=**/
  Divide1 : Product  Inputs=*/
  Divide{2..3,10..11} (4 alike) : Product  Inputs=**
  Divide8 : Product  Inputs=*/
  Divide9 : Product  Inputs=***
  Gain1 : Gain  Gain=1/5252.113
  Gain15 : Gain  Gain=1/MWS.Shaft.PGB.Ring.GR_gb %GR_gb = Ngb/Nem
  Gain4 : Gain  Gain=1/5252.113
  Gain5 : Gain  Gain=1/MWS.Shaft.PGB.Carrier.GR_gb %GR_gb = Ngb/Nem
  MinMax : MinMax
  MinMax2 : MinMax
  Mux1 : Mux  Inputs=3
  Mux3 : Mux  Inputs=3
  PwrMax_Base : Constant  Value=MWS.Cntrl.EMR.PwrMax_TEEM
  PwrMax_Base2 : Constant  Value=MWS.Cntrl.EMC.PwrMax_TEEM
  Sign : Signum
  Sign2 : Signum
  Sum1 : Sum  Inputs=|-+
  TrqMax_Base : Constant  Value=MWS.Cntrl.EMR.TrqMax_TEEM
  TrqMax_Base2 : Constant  Value=MWS.Cntrl.EMC.TrqMax_TEEM
  Zero : Constant  Value=0
  Zero1 : Constant  Value=0
  PemS_TEEM : Outport
  PemR_TEEM : Outport  Port=2
  PemC_TEEM : Outport  Port=3
  PemP_TEEM : Outport  Port=4
  wires:
  TrqMax_Base/1 -> Divide3/1
  Divide3/1 -> Gain1/1
  Divide1/1 -> Divide/2
  Abs/1 -> MinMax/1
  Gain5/1 -> Divide10/2
  PwrMax_Base2/1 -> Mux3/2
  Zero1/1 -> PemS_TEEM/1
  [NC] -> Gain5/1, Divide8/1
  Mux3/1 -> Abs2/1
  Divide/1 -> Mux1/1, Sign/1  "Power to LP from Coupling"
  MinMax/1 -> Divide2/2
  TrqMax_Base2/1 -> Divide10/1
  Divide10/1 -> Gain4/1
  Divide2/1 -> [PemR_Base], PemR_TEEM/1
  [NR] -> Gain15/1
  [PemR_Base] -> Divide9/1
  Gain4/1 -> Mux3/3
  Divide8/1 -> Divide9/2
  Pwr_TEEM/1 -> [Pwr_TEEM], Divide/1
  Gain1/1 -> Mux1/3
  Sum1/1 -> Mux3/1, Sign2/1
  [NR] -> Divide8/2
  Gain15/1 -> Divide3/2
  Abs2/1 -> MinMax2/1
  NC/1 -> [NC], Divide1/2
  PwrMax_Base/1 -> Mux1/2
  Mux1/1 -> Abs/1
  Divide11/1 -> PemC_TEEM/1
  NR/1 -> Divide1/1, [NR]
  MinMax2/1 -> Divide11/2
  Sign/1 -> Divide2/1
  CTrqCR/1 -> Divide9/3
  Sign2/1 -> Divide11/1
  CTrqCR1/1 -> Divide/3
  Divide9/1 -> Sum1/1
  [Pwr_TEEM] -> Sum1/2
  Zero/1 -> PemP_TEEM/1

== system AGTF30SysDyn_PExPIn/Control System/Electric Machine Controllers/VEATE EM Controllers/TEEM Power/TEEM Power/TEEM - HR LC CS  ==
  note: HP EM
  note: LP EM
  note: HP - RING, LP - CARRIER, COUPLING - SUN
  note: COUPLING EM
  Pwr_TEEM : Inport
  NS : Inport  Port=2
  NR : Inport  Port=3
  Abs : Abs
  Abs2 : Abs
  CTrqRS : Constant  Value=MWS.Shaft.PGB.TrqCoeff.CTrqRS
  CTrqRS1 : Constant  Value=MWS.Shaft.PGB.TrqCoeff.CTrqRS
  Divide : Product  Inputs=**/
  Divide1 : Product  Inputs=*/
  Divide{2..3,10..11} (4 alike) : Product  Inputs=**
  Divide8 : Product  Inputs=*/
  Divide9 : Product  Inputs=***
  Gain1 : Gain  Gain=1/5252.113
  Gain15 : Gain  Gain=1/MWS.Shaft.PGB.Sun.GR_gb %GR_gb = Ngb/Nem
  Gain4 : Gain  Gain=1/5252.113
  Gain5 : Gain  Gain=1/MWS.Shaft.PGB.Ring.GR_gb %GR_gb = Ngb/Nem
  MinMax : MinMax
  MinMax2 : MinMax
  Mux1 : Mux  Inputs=3
  Mux3 : Mux  Inputs=3
  PwrMax_Base : Constant  Value=MWS.Cntrl.EMS.PwrMax_TEEM
  PwrMax_Base2 : Constant  Value=MWS.Cntrl.EMR.PwrMax_TEEM
  Sign : Signum
  Sign2 : Signum
  Sum1 : Sum  Inputs=|-+
  TrqMax_Base : Constant  Value=MWS.Cntrl.EMS.TrqMax_TEEM
  TrqMax_Base2 : Constant  Value=MWS.Cntrl.EMR.TrqMax_TEEM
  Zero : Constant  Value=0
  Zero1 : Constant  Value=0
  PemS_TEEM : Outport
  PemR_TEEM : Outport  Port=2
  PemC_TEEM : Outport  Port=3
  PemP_TEEM : Outport  Port=4
  wires:
  Zero/1 -> PemP_TEEM/1
  [Pwr_TEEM] -> Sum1/2
  Divide9/1 -> Sum1/1
  CTrqRS1/1 -> Divide/3
  Sign2/1 -> Divide11/1
  CTrqRS/1 -> Divide9/3
  Sign/1 -> Divide2/1
  MinMax2/1 -> Divide11/2
  NS/1 -> [NS], Divide1/1
  Divide11/1 -> PemR_TEEM/1
  Mux1/1 -> Abs/1
  PwrMax_Base/1 -> Mux1/2
  NR/1 -> [NR], Divide1/2
  Abs2/1 -> MinMax2/1
  Gain15/1 -> Divide3/2
  [NS] -> Divide8/2
  Sum1/1 -> Sign2/1, Mux3/1
  Gain1/1 -> Mux1/3
  Pwr_TEEM/1 -> Divide/1, [Pwr_TEEM]
  Divide8/1 -> Divide9/2
  Gain4/1 -> Mux3/3
  [PemS_Base] -> Divide9/1
  [NS] -> Gain15/1
  Divide2/1 -> [PemS_Base], PemS_TEEM/1
  Divide10/1 -> Gain4/1
  TrqMax_Base2/1 -> Divide10/1
  MinMax/1 -> Divide2/2
  Divide/1 -> Sign/1, Mux1/1  "Power to LP from Coupling"
  Mux3/1 -> Abs2/1
  [NR] -> Divide8/1, Gain5/1
  Zero1/1 -> PemC_TEEM/1
  PwrMax_Base2/1 -> Mux3/2
  Gain5/1 -> Divide10/2
  Abs/1 -> MinMax/1
  Divide1/1 -> Divide/2
  Divide3/1 -> Gain1/1
  TrqMax_Base/1 -> Divide3/1

== system AGTF30SysDyn_PExPIn/Control System/Electric Machine Controllers/VEATE EM Controllers/TEEM Power/TEEM Power/TEEM - HR LS CC ==
  note: HP EM
  note: LP EM
  note: HP - RING, LP - SUN, COUPLING - CARRIER
  note: COUPLING EM
  Pwr_TEEM : Inport
  NR : Inport  Port=2
  NC : Inport  Port=3
  Abs : Abs
  Abs2 : Abs
  CTrqRC : Constant  Value=MWS.Shaft.PGB.TrqCoeff.CTrqRC
  CTrqRC1 : Constant  Value=MWS.Shaft.PGB.TrqCoeff.CTrqRC
  Divide : Product  Inputs=**/
  Divide1 : Product  Inputs=*/
  Divide{2..3,10..11} (4 alike) : Product  Inputs=**
  Divide8 : Product  Inputs=*/
  Divide9 : Product  Inputs=***
  Gain1 : Gain  Gain=1/5252.113
  Gain15 : Gain  Gain=1/MWS.Shaft.PGB.Carrier.GR_gb %GR_gb = Ngb/Nem
  Gain4 : Gain  Gain=1/5252.113
  Gain5 : Gain  Gain=1/MWS.Shaft.PGB.Ring.GR_gb %GR_gb = Ngb/Nem
  MinMax : MinMax
  MinMax2 : MinMax
  Mux1 : Mux  Inputs=3
  Mux3 : Mux  Inputs=3
  PwrMax_Base : Constant  Value=MWS.Cntrl.EMC.PwrMax_TEEM
  PwrMax_Base2 : Constant  Value=MWS.Cntrl.EMR.PwrMax_TEEM
  Sign : Signum
  Sign2 : Signum
  Sum1 : Sum  Inputs=|-+
  TrqMax_Base : Constant  Value=MWS.Cntrl.EMC.TrqMax_TEEM
  TrqMax_Base2 : Constant  Value=MWS.Cntrl.EMR.TrqMax_TEEM
  Zero : Constant  Value=0
  Zero1 : Constant  Value=0
  PemS_TEEM : Outport
  PemR_TEEM : Outport  Port=2
  PemC_TEEM : Outport  Port=3
  PemP_TEEM : Outport  Port=4
  wires:
  Zero/1 -> PemP_TEEM/1
  [Pwr_TEEM] -> Sum1/2
  Divide9/1 -> Sum1/1
  CTrqRC1/1 -> Divide/3
  Sign2/1 -> Divide11/1
  CTrqRC/1 -> Divide9/3
  Sign/1 -> Divide2/1
  MinMax2/1 -> Divide11/2
  NC/1 -> [NC], Divide1/1
  Divide11/1 -> PemR_TEEM/1
  Mux1/1 -> Abs/1
  PwrMax_Base/1 -> Mux1/2
  NR/1 -> Divide1/2, [NR]
  Abs2/1 -> MinMax2/1
  Gain15/1 -> Divide3/2
  [NC] -> Divide8/2
  Sum1/1 -> Sign2/1, Mux3/1
  Gain1/1 -> Mux1/3
  Pwr_TEEM/1 -> Divide/1, [Pwr_TEEM]
  Divide8/1 -> Divide9/2
  Gain4/1 -> Mux3/3
  [PemC_Base] -> Divide9/1
  [NC] -> Gain15/1
  Divide2/1 -> [PemC_Base], PemC_TEEM/1
  Divide10/1 -> Gain4/1
  TrqMax_Base2/1 -> Divide10/1
  MinMax/1 -> Divide2/2
  Divide/1 -> Sign/1, Mux1/1  "Power to LP from Coupling"
  Mux3/1 -> Abs2/1
  [NR] -> Divide8/1, Gain5/1
  Zero1/1 -> PemS_TEEM/1
  PwrMax_Base2/1 -> Mux3/2
  Gain5/1 -> Divide10/2
  Abs/1 -> MinMax/1
  Divide1/1 -> Divide/2
  Divide3/1 -> Gain1/1
  TrqMax_Base/1 -> Divide3/1

== system AGTF30SysDyn_PExPIn/Control System/Electric Machine Controllers/VEATE EM Controllers/TEEM Power/TEEM Power/TEEM - HS LC CR ==
  note: COUPLING EM
  note: HP - SUN, LP - CARRIER, COUPLING - RING
  note: LP EM
  note: HP EM
  Pwr_TEEM : Inport
  NS : Inport  Port=2
  NR : Inport  Port=3
  Abs : Abs
  Abs2 : Abs
  CTrqSR : Constant  Value=MWS.Shaft.PGB.TrqCoeff.CTrqSR
  CTrqSR1 : Constant  Value=MWS.Shaft.PGB.TrqCoeff.CTrqSR
  Divide : Product  Inputs=**/
  Divide1 : Product  Inputs=*/
  Divide{2..3,10..11} (4 alike) : Product  Inputs=**
  Divide8 : Product  Inputs=*/
  Divide9 : Product  Inputs=***
  Gain1 : Gain  Gain=1/5252.113
  Gain15 : Gain  Gain=1/MWS.Shaft.PGB.Ring.GR_gb %GR_gb = Ngb/Nem
  Gain4 : Gain  Gain=1/5252.113
  Gain5 : Gain  Gain=1/MWS.Shaft.PGB.Sun.GR_gb %GR_gb = Ngb/Nem
  MinMax : MinMax
  MinMax2 : MinMax
  Mux1 : Mux  Inputs=3
  Mux3 : Mux  Inputs=3
  PwrMax_Base : Constant  Value=MWS.Cntrl.EMR.PwrMax_TEEM
  PwrMax_Base2 : Constant  Value=MWS.Cntrl.EMS.PwrMax_TEEM  VectorParams1D=off
  Sign : Signum
  Sign2 : Signum
  Sum1 : Sum  Inputs=|-+
  TrqMax_Base : Constant  Value=MWS.Cntrl.EMR.TrqMax_TEEM
  TrqMax_Base2 : Constant  Value=MWS.Cntrl.EMS.TrqMax_TEEM
  Zero : Constant  Value=0
  zero : Constant  Value=0
  PemS_TEEM : Outport
  PemR_TEEM : Outport  Port=2
  PemC_TEEM : Outport  Port=3
  PemP_TEEM : Outport  Port=4
  wires:
  TrqMax_Base/1 -> Divide3/1
  Divide3/1 -> Gain1/1
  Divide1/1 -> Divide/2
  Abs/1 -> MinMax/1
  Gain5/1 -> Divide10/2
  PwrMax_Base2/1 -> Mux3/2
  zero/1 -> PemC_TEEM/1
  [NS] -> Gain5/1, Divide8/1
  Mux3/1 -> Abs2/1
  Divide/1 -> Mux1/1, Sign/1  "Power to LP from Coupling"
  MinMax/1 -> Divide2/2
  TrqMax_Base2/1 -> Divide10/1
  Divide10/1 -> Gain4/1
  Divide2/1 -> PemR_TEEM/1, [PemR_Base]
  [NR] -> Gain15/1
  [PemR_Base] -> Divide9/1
  Gain4/1 -> Mux3/3
  Divide8/1 -> Divide9/2
  Pwr_TEEM/1 -> [Pwr_TEEM], Divide/1
  Gain1/1 -> Mux1/3
  Sum1/1 -> Mux3/1, Sign2/1
  [NR] -> Divide8/2
  Gain15/1 -> Divide3/2
  Abs2/1 -> MinMax2/1
  NS/1 -> Divide1/2, [NS]
  PwrMax_Base/1 -> Mux1/2
  Mux1/1 -> Abs/1
  Divide11/1 -> PemS_TEEM/1
  NR/1 -> Divide1/1, [NR]
  MinMax2/1 -> Divide11/2
  Sign/1 -> Divide2/1
  CTrqSR/1 -> Divide9/3
  Sign2/1 -> Divide11/1
  CTrqSR1/1 -> Divide/3
  Divide9/1 -> Sum1/1
  [Pwr_TEEM] -> Sum1/2
  Zero/1 -> PemP_TEEM/1

== system AGTF30SysDyn_PExPIn/Control System/Electric Machine Controllers/VEATE EM Controllers/TEEM Power/TEEM Power/TEEM- HS LR CC ==
  note: HP EM
  note: LP EM
  note: HP - SUN, LP - RING, COUPLING - CARRIER
  note: COUPLING EM
  Pwr_TEEM : Inport
  NS : Inport  Port=2
  NC : Inport  Port=3
  Abs : Abs
  Abs2 : Abs
  CTrqSC : Constant  Value=MWS.Shaft.PGB.TrqCoeff.CTrqSC
  CTrqSC1 : Constant  Value=MWS.Shaft.PGB.TrqCoeff.CTrqSC
  Divide : Product  Inputs=**/
  Divide1 : Product  Inputs=*/
  Divide{2..3,10..11} (4 alike) : Product  Inputs=**
  Divide8 : Product  Inputs=*/
  Divide9 : Product  Inputs=***
  Gain1 : Gain  Gain=1/5252.113
  Gain15 : Gain  Gain=1/MWS.Shaft.PGB.Carrier.GR_gb %GR_gb = Ngb/Nem
  Gain4 : Gain  Gain=1/5252.113
  Gain5 : Gain  Gain=1/MWS.Shaft.PGB.Sun.GR_gb %GR_gb = Ngb/Nem
  MinMax : MinMax
  MinMax2 : MinMax
  Mux1 : Mux  Inputs=3
  Mux3 : Mux  Inputs=3
  PwrMax_Base : Constant  Value=MWS.Cntrl.EMC.PwrMax_TEEM
  PwrMax_Base2 : Constant  Value=MWS.Cntrl.EMS.PwrMax_TEEM
  Sign : Signum
  Sign2 : Signum
  Sum1 : Sum  Inputs=|-+
  TrqMax_Base : Constant  Value=MWS.Cntrl.EMC.TrqMax_TEEM
  TrqMax_Base2 : Constant  Value=MWS.Cntrl.EMS.TrqMax_TEEM
  Zero : Constant  Value=0
  Zero1 : Constant  Value=0
  PemS_TEEM : Outport
  PemR_TEEM : Outport  Port=2
  PemC_TEEM : Outport  Port=3
  PemP_TEEM : Outport  Port=4
  wires:
  Zero/1 -> PemP_TEEM/1
  Divide9/1 -> Sum1/1
  CTrqSC/1 -> Divide/3
  Sign2/1 -> Divide11/1
  CTrqSC1/1 -> Divide9/3
  Sign/1 -> Divide2/1
  MinMax2/1 -> Divide11/2
  NC/1 -> Divide1/1, [NC]
  Divide11/1 -> PemS_TEEM/1
  Mux1/1 -> Abs/1
  PwrMax_Base/1 -> Mux1/2
  NS/1 -> [NS], Divide1/2
  Abs2/1 -> MinMax2/1
  Gain15/1 -> Divide3/2
  [NC] -> Divide8/2
  Sum1/1 -> Sign2/1, Mux3/1
  Gain1/1 -> Mux1/3
  Pwr_TEEM/1 -> Divide/1, [Pwr_TEEM]
  Divide8/1 -> Divide9/2
  Gain4/1 -> Mux3/3
  [PemC_TEEM] -> Divide9/1
  [NC] -> Gain15/1
  Divide2/1 -> [PemC_TEEM], PemC_TEEM/1
  Divide10/1 -> Gain4/1
  TrqMax_Base2/1 -> Divide10/1
  MinMax/1 -> Divide2/2
  Divide/1 -> Sign/1, Mux1/1  "Power to LP from Coupling"
  Mux3/1 -> Abs2/1
  [NS] -> Divide8/1, Gain5/1
  Zero1/1 -> PemR_TEEM/1
  PwrMax_Base2/1 -> Mux3/2
  Gain5/1 -> Divide10/2
  Abs/1 -> MinMax/1
  Divide1/1 -> Divide/2
  Divide3/1 -> Gain1/1
  TrqMax_Base/1 -> Divide3/1
  [Pwr_TEEM] -> Sum1/2
